simulink model "Devastator_simulator_2019a"  (R2019a)
settings: Solver=ode1  StartTime=0.0  StopTime=90  FixedStep=0.01  RelTol=1e-3
values from neighbouring files (symbols this model uses):
  Kd_psi = 0    [Devastator_simulator.m]
  Kd_Vx = 0    [Devastator_simulator.m]
  Ki_psi = 0    [Devastator_simulator.m]
  Ki_Vx = 1.85    [Devastator_simulator.m]
  Kp_psi = 0.4    [Devastator_simulator.m]
  Kp_Vx = 2    [Devastator_simulator.m]
  ox = str2num(x{6})    [Devastator_simulator.m]
  oy = str2num(x{7})    [Devastator_simulator.m]
  psi_0 = str2num(x{5})/180*pi    [Devastator_simulator.m]
  X_0 = str2num(x{3})    [Devastator_simulator.m]
  X_goal = str2num(x{1})    [Devastator_simulator.m]
  Y_0 = str2num(x{4})    [Devastator_simulator.m]
  Y_goal = str2num(x{2})    [Devastator_simulator.m]
libraries: simulink x4, slident x1
settings Model: Creator=PC  LastModifiedBy=PC

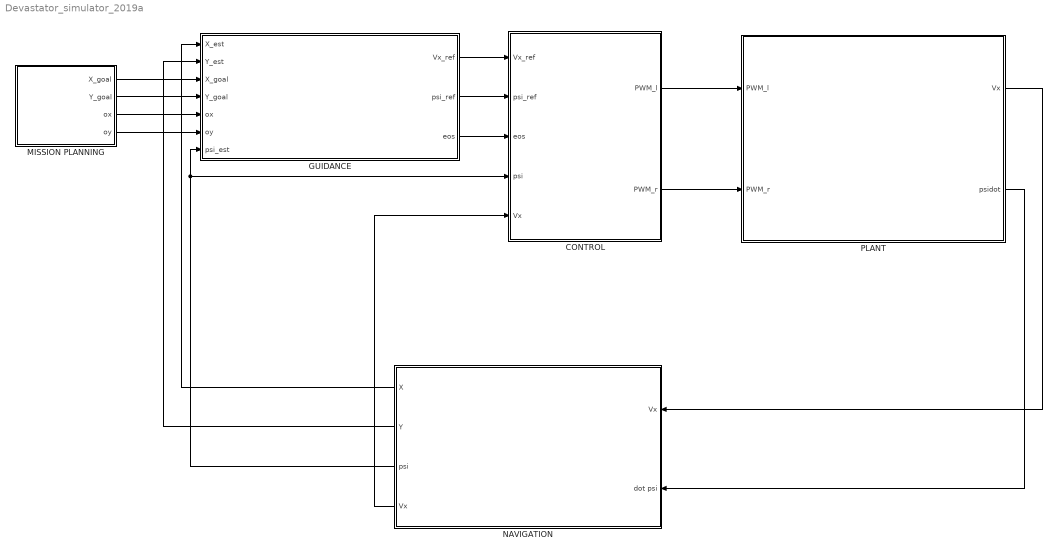
== system Devastator_simulator_2019a ==
  "CONTROL " : Subsystem
  "GUIDANCE " : Subsystem
  MISSION PLANNING : Subsystem
  NAVIGATION : Subsystem
  PLANT : Subsystem
  wires:
  "CONTROL "/1(PWM_l) -> PLANT/1(PWM_l)
  "CONTROL "/2(PWM_r) -> PLANT/2(PWM_r)
  PLANT/1(Vx) -> NAVIGATION/1(Vx)
  PLANT/2(psidot) -> NAVIGATION/2(dot psi)
  "GUIDANCE "/3(eos) -> "CONTROL "/3(eos)
  "GUIDANCE "/2(psi_ref) -> "CONTROL "/2(psi_ref)
  "GUIDANCE "/1(Vx_ref) -> "CONTROL "/1(Vx_ref)
  MISSION PLANNING/4(oy) -> "GUIDANCE "/6(oy)
  MISSION PLANNING/3(ox) -> "GUIDANCE "/5(ox)
  MISSION PLANNING/2(Y_goal) -> "GUIDANCE "/4(Y_goal)
  MISSION PLANNING/1(X_goal) -> "GUIDANCE "/3(X_goal)
  NAVIGATION/2(Y) -> "GUIDANCE "/2(Y_est)
  NAVIGATION/1(X) -> "GUIDANCE "/1(X_est)
  NAVIGATION/4(" Vx") -> "CONTROL "/5(Vx)
  NAVIGATION/3(psi) -> "GUIDANCE "/7(psi_est), "CONTROL "/4(psi)

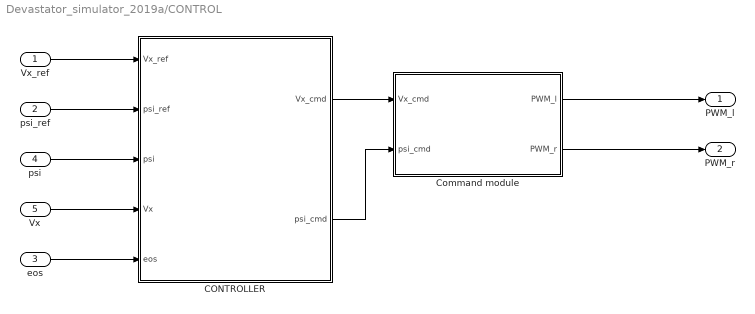
== system Devastator_simulator_2019a/CONTROL  ==
  Vx_ref : Inport
  psi_ref : Inport  Port=2
  eos : Inport  Port=3
  psi : Inport  Port=4
  Vx : Inport  Port=5
  CONTROLLER : Subsystem
  Command module : Subsystem
  PWM_l : Outport
  PWM_r : Outport  Port=2
  wires:
  psi_ref/1 -> CONTROLLER/2(psi_ref)
  eos/1 -> CONTROLLER/5(eos)
  psi/1 -> CONTROLLER/3(psi)
  CONTROLLER/1(Vx_cmd) -> Command module/1(Vx_cmd)
  CONTROLLER/2(psi_cmd) -> Command module/2(psi_cmd)
  Vx/1 -> CONTROLLER/4(Vx)
  Vx_ref/1 -> CONTROLLER/1(Vx_ref)
  Command module/1(PWM_l) -> PWM_l/1
  Command module/2(PWM_r) -> PWM_r/1

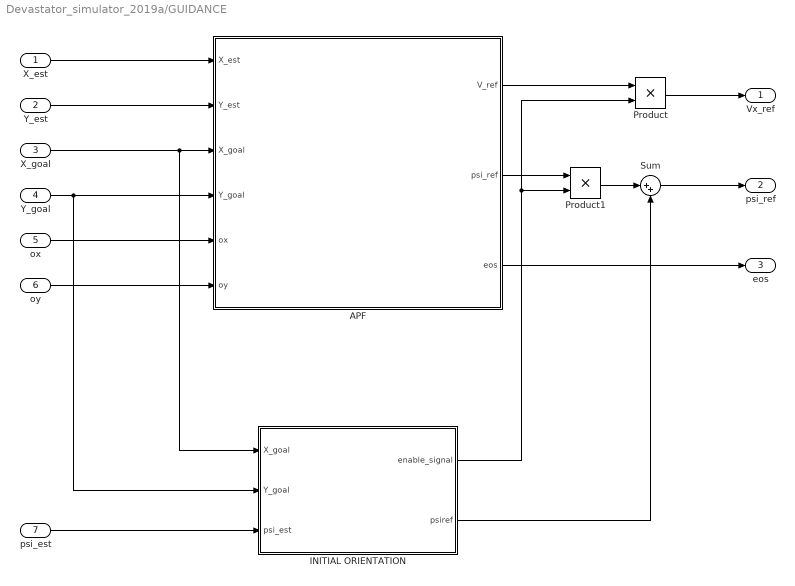
== system Devastator_simulator_2019a/GUIDANCE  ==
  X_est : Inport
  Y_est : Inport  Port=2
  X_goal : Inport  Port=3
  Y_goal : Inport  Port=4
  ox : Inport  Port=5
  oy : Inport  Port=6
  psi_est : Inport  Port=7
  APF : Subsystem
  INITIAL ORIENTATION : Subsystem
  Product : Product
  Product1 : Product
  Sum : Sum  Inputs=|++
  Vx_ref : Outport
  psi_ref : Outport  Port=2
  eos : Outport  Port=3
  wires:
  X_goal/1 -> INITIAL ORIENTATION/1(X_goal), APF/3(X_goal)
  Y_goal/1 -> INITIAL ORIENTATION/2(Y_goal), APF/4(Y_goal)
  X_est/1 -> APF/1(X_est)
  Y_est/1 -> APF/2(Y_est)
  ox/1 -> APF/5(ox)
  oy/1 -> APF/6(oy)
  Sum/1 -> psi_ref/1
  psi_est/1 -> INITIAL ORIENTATION/3(psi_est)
  INITIAL ORIENTATION/2(psiref) -> Sum/2
  APF/1(V_ref) -> Product/1
  Product/1 -> Vx_ref/1
  INITIAL ORIENTATION/1(enable_signal) -> Product1/2, Product/2
  APF/2(psi_ref) -> Product1/1
  Product1/1 -> Sum/1
  APF/3(eos) -> eos/1

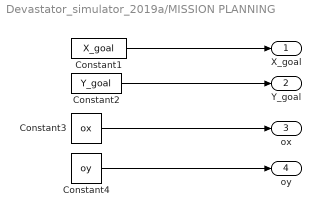
== system Devastator_simulator_2019a/MISSION PLANNING ==
  Constant1 : Constant  Value=X_goal
  Constant2 : Constant  Value=Y_goal
  Constant3 : Constant  Value=ox
  Constant4 : Constant  Value=oy
  X_goal : Outport
  Y_goal : Outport  Port=2
  ox : Outport  Port=3
  oy : Outport  Port=4
  wires:
  Constant4/1 -> oy/1
  Constant3/1 -> ox/1
  Constant2/1 -> Y_goal/1
  Constant1/1 -> X_goal/1

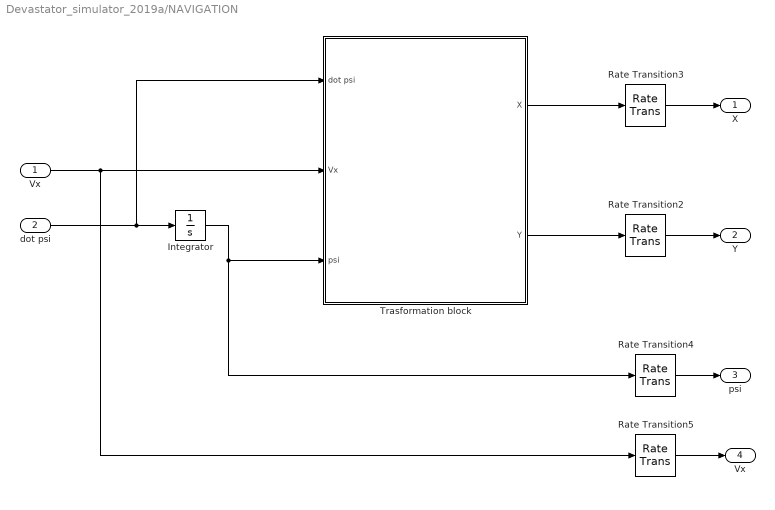
== system Devastator_simulator_2019a/NAVIGATION ==
  Vx : Inport
  dot psi : Inport  Port=2
  Integrator : Integrator  InitialCondition=psi_0  WrapState=on
  Rate Transition{2..5} (4 alike) : RateTransition  OutPortSampleTime=0.1
  Trasformation block : Subsystem
  X : Outport
  Y : Outport  Port=2
  psi : Outport  Port=3
  " Vx" : Outport  Port=4
  wires:
  dot psi/1 -> Trasformation block/1(dot psi), Integrator/1
  Rate Transition5/1 -> " Vx"/1
  Trasformation block/1(X) -> Rate Transition3/1
  Trasformation block/2(Y) -> Rate Transition2/1
  Rate Transition4/1 -> psi/1
  Rate Transition2/1 -> Y/1
  Vx/1 -> Rate Transition5/1, Trasformation block/2(Vx)
  Rate Transition3/1 -> X/1
  Integrator/1 -> Rate Transition4/1, Trasformation block/3(psi)

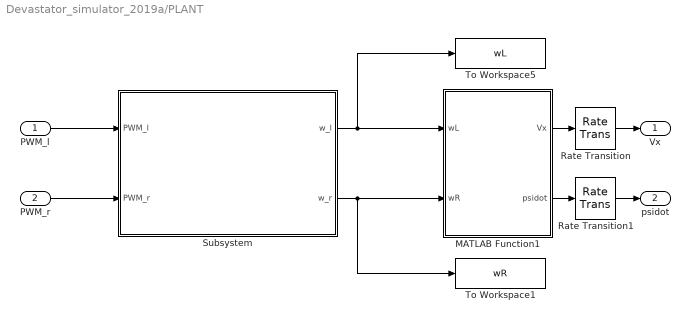
== system Devastator_simulator_2019a/PLANT ==
  PWM_l : Inport
  PWM_r : Inport  Port=2
  MATLAB Function1 : MATLAB Function  TreatAsAtomicUnit=on
  Rate Transition : RateTransition
  Rate Transition1 : RateTransition
  Subsystem : Subsystem
  To Workspace1 : ToWorkspace  VariableName=wR  SaveFormat=Structure With Time  SampleTime=-1
  To Workspace5 : ToWorkspace  VariableName=wL  SaveFormat=Structure With Time  SampleTime=-1
  Vx : Outport
  psidot : Outport  Port=2
  wires:
  MATLAB Function1/1(Vx) -> Rate Transition/1
  MATLAB Function1/2(psidot) -> Rate Transition1/1
  Subsystem/2(w_r) -> To Workspace1/1, MATLAB Function1/2(wR)
  Subsystem/1(w_l) -> To Workspace5/1, MATLAB Function1/1(wL)
  PWM_l/1 -> Subsystem/1(PWM_l)
  PWM_r/1 -> Subsystem/2(PWM_r)
  Rate Transition/1 -> Vx/1
  Rate Transition1/1 -> psidot/1

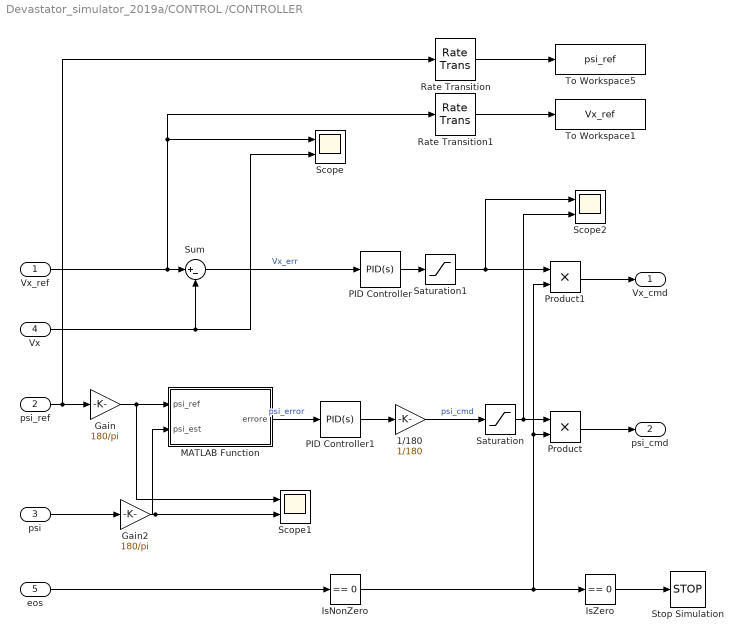
== system Devastator_simulator_2019a/CONTROL /CONTROLLER ==
  Vx_ref : Inport
  psi_ref : Inport  Port=2
  psi : Inport  Port=3
  Vx : Inport  Port=4
  eos : Inport  Port=5
  1/180 : Gain  Gain=1/180
  Gain : Gain  Gain=180/pi
  Gain2 : Gain  Gain=180/pi
  IsNonZero : simulink/Logic and Bit Operations/Compare To Zero  relop===  OutDataTypeStr=boolean
  IsZero : simulink/Logic and Bit Operations/Compare To Zero  relop===  OutDataTypeStr=boolean
  MATLAB Function : MATLAB Function  TreatAsAtomicUnit=on
  PID Controller : simulink/Continuous/PID Controller  Controller=PID  Form=Parallel  TimeDomain=Continuous-time  SampleTime=-1  IntegratorMethod=Forward Euler  FilterMethod=Forward Euler  ControllerParametersSource=internal  P=Kp_Vx  I=Ki_Vx  D=Kd_Vx  UseFilter=on  N=100  TunerSelectOption=Transfer Function Based (PID Tuner App)  InitialConditionSource=internal  InitialConditionForIntegrator=0  InitialConditionForFilter=0  DifferentiatorICPrevScaledInput=0  ExternalReset=none  TrackingMode=off  Kt=1  LimitOutput=off  UpperSaturationLimit=inf  LowerSaturationLimit=-inf  LinearizeAsGain=on  AntiWindupMode=none  Kb=1  POutMin=[]  POutMax=[]  IOutMin=[]  IOutMax=[]  DOutMin=[]  DOutMax=[]  NOutMin=[]  NOutMax=[]  SumOutMin=[]  SumOutMax=[]  SaturationOutMin=[]  SaturationOutMax=[]  PParamMin=[]  PParamMax=[]  IParamMin=[]  IParamMax=[]  DParamMin=[]  DParamMax=[]  NParamMin=[]  NParamMax=[]  KbParamMin=[]  KbParamMax=[]  KtParamMin=[]  KtParamMax=[]  KbOutMin=[]  KbOutMax=[]  KtOutMin=[]  KtOutMax=[]  IntegratorOutMin=[]  IntegratorOutMax=[]  FilterOutMin=[]  FilterOutMax=[]  SumI1OutMin=[]  SumI1OutMax=[]  SumI2OutMin=[]  SumI2OutMax=[]  SumI3OutMin=[]  SumI3OutMax=[]  SumI4OutMin=[]  SumI4OutMax=[]  SumDOutMin=[]  SumDOutMax=[]  DifferentiatorOutMin=[]  DifferentiatorOutMax=[]  FilterDiffOutCoefMin=[]  FilterDiffOutCoefMax=[]  ReciprocalOutMin=[]  ReciprocalOutMax=[]  SumDenOutMin=[]  SumDenOutMax=[]  SumNumOutMin=[]  SumNumOutMax=[]  DivideOutMin=[]  DivideOutMax=[]  IntegratorContinuousStateAttributes=''  IntegratorStateMustResolveToSignalObject=off  IntegratorRTWStateStorageClass=Auto  FilterContinuousStateAttributes=''  FilterStateMustResolveToSignalObject=off  FilterRTWStateStorageClass=Auto  ParallelPVariant=InternalParameters  IdealPVariant=Disabled  IVariant=InternalParameters  DVariant=InternalParameters  IntegratorVariant=Continuous  SatVariant=Disabled  AWVariant=Passthrough  PCopyVariant=Disabled  TRVariant=Disabled  FdbkBlocksVariant=Forward  IdealPFdbkVariant=Disabled  SatFdbkVariant=Disabled  DerivativeFilterVariant=ContFilter  NVariant=InternalParameters  NCopyVariant=Disabled  FilterICVariant=InternalICsFilter  IntegratorICVariant=InternalICs  ExternalResetVariant=Disabled  TRSumVariant=Passthrough  SumFdbkVariant=Disabled  SumVariant=Sum_PID
  PID Controller1 : simulink/Continuous/PID Controller  Controller=PID  Form=Parallel  TimeDomain=Continuous-time  SampleTime=-1  IntegratorMethod=Forward Euler  FilterMethod=Forward Euler  ControllerParametersSource=internal  P=Kp_psi  I=Ki_psi  D=Kd_psi  UseFilter=on  N=100  TunerSelectOption=Transfer Function Based (PID Tuner App)  InitialConditionSource=internal  InitialConditionForIntegrator=0  InitialConditionForFilter=0  DifferentiatorICPrevScaledInput=0  ExternalReset=none  TrackingMode=off  Kt=1  LimitOutput=off  UpperSaturationLimit=inf  LowerSaturationLimit=-inf  LinearizeAsGain=on  AntiWindupMode=none  Kb=1  POutMin=[]  POutMax=[]  IOutMin=[]  IOutMax=[]  DOutMin=[]  DOutMax=[]  NOutMin=[]  NOutMax=[]  SumOutMin=[]  SumOutMax=[]  SaturationOutMin=[]  SaturationOutMax=[]  PParamMin=[]  PParamMax=[]  IParamMin=[]  IParamMax=[]  DParamMin=[]  DParamMax=[]  NParamMin=[]  NParamMax=[]  KbParamMin=[]  KbParamMax=[]  KtParamMin=[]  KtParamMax=[]  KbOutMin=[]  KbOutMax=[]  KtOutMin=[]  KtOutMax=[]  IntegratorOutMin=[]  IntegratorOutMax=[]  FilterOutMin=[]  FilterOutMax=[]  SumI1OutMin=[]  SumI1OutMax=[]  SumI2OutMin=[]  SumI2OutMax=[]  SumI3OutMin=[]  SumI3OutMax=[]  SumI4OutMin=[]  SumI4OutMax=[]  SumDOutMin=[]  SumDOutMax=[]  DifferentiatorOutMin=[]  DifferentiatorOutMax=[]  FilterDiffOutCoefMin=[]  FilterDiffOutCoefMax=[]  ReciprocalOutMin=[]  ReciprocalOutMax=[]  SumDenOutMin=[]  SumDenOutMax=[]  SumNumOutMin=[]  SumNumOutMax=[]  DivideOutMin=[]  DivideOutMax=[]  IntegratorContinuousStateAttributes=''  IntegratorStateMustResolveToSignalObject=off  IntegratorRTWStateStorageClass=Auto  FilterContinuousStateAttributes=''  FilterStateMustResolveToSignalObject=off  FilterRTWStateStorageClass=Auto  ParallelPVariant=InternalParameters  IdealPVariant=Disabled  IVariant=InternalParameters  DVariant=InternalParameters  IntegratorVariant=Continuous  SatVariant=Disabled  AWVariant=Passthrough  PCopyVariant=Disabled  TRVariant=Disabled  FdbkBlocksVariant=Forward  IdealPFdbkVariant=Disabled  SatFdbkVariant=Disabled  DerivativeFilterVariant=ContFilter  NVariant=InternalParameters  NCopyVariant=Disabled  FilterICVariant=InternalICsFilter  IntegratorICVariant=InternalICs  ExternalResetVariant=Disabled  TRSumVariant=Passthrough  SumFdbkVariant=Disabled  SumVariant=Sum_PID
  Product : Product
  Product1 : Product
  Rate Transition : RateTransition
  Rate Transition1 : RateTransition
  Saturation : Saturate
  Saturation1 : Saturate  UpperLimit=1  LowerLimit=-1
  Scope : Scope  NumInputPorts=2
  Scope1 : Scope  NumInputPorts=2
  Scope2 : Scope  NumInputPorts=2
  Stop Simulation : Stop
  Sum : Sum  Inputs=|+-
  To Workspace1 : ToWorkspace  VariableName=Vx_ref  SaveFormat=Structure With Time  SampleTime=-1
  To Workspace5 : ToWorkspace  VariableName=psi_ref  SaveFormat=Structure With Time  SampleTime=-1
  Vx_cmd : Outport
  psi_cmd : Outport  Port=2
  wires:
  MATLAB Function/1(errore) -> PID Controller1/1  "psi_error"
  1/180/1 -> Saturation/1  "psi_cmd"
  PID Controller/1 -> Saturation1/1
  PID Controller1/1 -> 1/180/1
  Gain/1 -> Scope1/1, MATLAB Function/1(psi_ref)
  Vx_ref/1 -> Rate Transition1/1, Scope/1, Sum/1
  Vx/1 -> Scope/2, Sum/2
  Gain2/1 -> Scope1/2, MATLAB Function/2(psi_est)
  eos/1 -> IsNonZero/1
  Saturation/1 -> Scope2/2, Product/1
  Product/1 -> psi_cmd/1
  Saturation1/1 -> Scope2/1, Product1/1
  Product1/1 -> Vx_cmd/1
  IsNonZero/1 -> IsZero/1, Product1/2, Product/2
  IsZero/1 -> Stop Simulation/1
  psi_ref/1 -> Rate Transition/1, Gain/1
  psi/1 -> Gain2/1
  Rate Transition/1 -> To Workspace5/1
  Rate Transition1/1 -> To Workspace1/1
  Sum/1 -> PID Controller/1  "Vx_err"

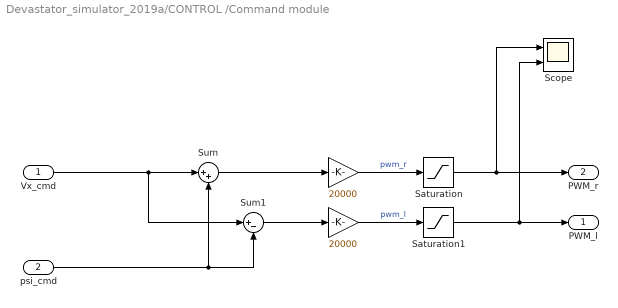
== system Devastator_simulator_2019a/CONTROL /Command module ==
  Vx_cmd : Inport
  psi_cmd : Inport  Port=2
  " " : Gain  Gain=20000
  "   " : Gain  Gain=20000
  Saturation : Saturate  UpperLimit=20000  LowerLimit=-20000
  Saturation1 : Saturate  UpperLimit=20000  LowerLimit=-20000
  Scope : Scope  NumInputPorts=2
  Sum : Sum  Inputs=|++
  Sum1 : Sum  Inputs=|+-
  PWM_l : Outport
  PWM_r : Outport  Port=2
  wires:
  "   "/1 -> Saturation1/1  "pwm_l"
  Sum1/1 -> "   "/1
  Vx_cmd/1 -> Sum/1, Sum1/1
  psi_cmd/1 -> Sum1/2, Sum/2
  Sum/1 -> " "/1
  " "/1 -> Saturation/1  "pwm_r"
  Saturation/1 -> Scope/1, PWM_r/1
  Saturation1/1 -> Scope/2, PWM_l/1

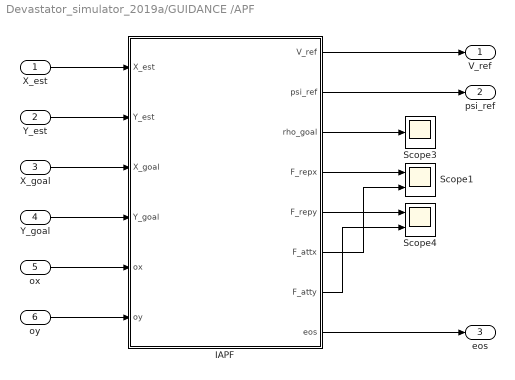
== system Devastator_simulator_2019a/GUIDANCE /APF ==
  X_est : Inport
  Y_est : Inport  Port=2
  X_goal : Inport  Port=3
  Y_goal : Inport  Port=4
  ox : Inport  Port=5
  oy : Inport  Port=6
  IAPF : MATLAB Function  TreatAsAtomicUnit=on
  Scope1 : Scope  NumInputPorts=2
  Scope3 : Scope
  Scope4 : Scope  NumInputPorts=2
  V_ref : Outport
  psi_ref : Outport  Port=2
  eos : Outport  Port=3
  wires:
  IAPF/1(V_ref) -> V_ref/1
  IAPF/6(F_attx) -> Scope1/2
  IAPF/3(rho_goal) -> Scope3/1
  IAPF/4(F_repx) -> Scope1/1
  IAPF/7(F_atty) -> Scope4/2
  IAPF/5(F_repy) -> Scope4/1
  X_est/1 -> IAPF/1(X_est)
  ox/1 -> IAPF/5(ox)
  IAPF/2(psi_ref) -> psi_ref/1
  Y_est/1 -> IAPF/2(Y_est)
  oy/1 -> IAPF/6(oy)
  IAPF/8(eos) -> eos/1
  X_goal/1 -> IAPF/3(X_goal)
  Y_goal/1 -> IAPF/4(Y_goal)

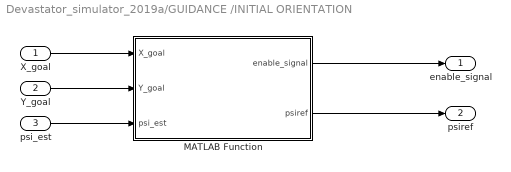
== system Devastator_simulator_2019a/GUIDANCE /INITIAL ORIENTATION ==
  X_goal : Inport
  Y_goal : Inport  Port=2
  psi_est : Inport  Port=3
  MATLAB Function : MATLAB Function  TreatAsAtomicUnit=on
  enable_signal : Outport
  psiref : Outport  Port=2
  wires:
  psi_est/1 -> MATLAB Function/3(psi_est)
  MATLAB Function/2(psiref) -> psiref/1
  Y_goal/1 -> MATLAB Function/2(Y_goal)
  X_goal/1 -> MATLAB Function/1(X_goal)
  MATLAB Function/1(enable_signal) -> enable_signal/1

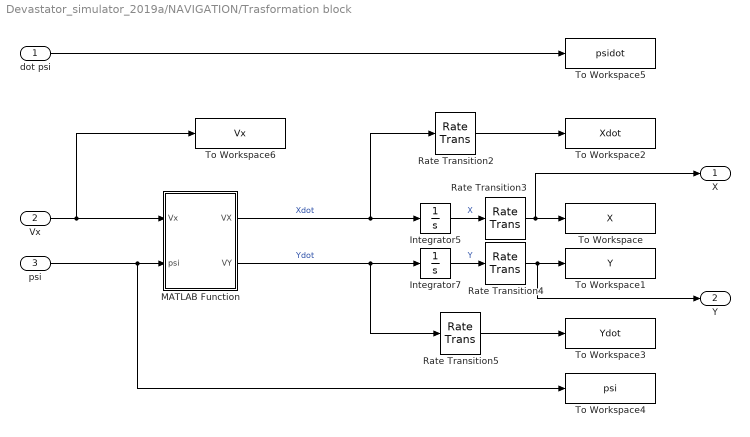
== system Devastator_simulator_2019a/NAVIGATION/Trasformation block ==
  dot psi : Inport
  Vx : Inport  Port=2
  psi : Inport  Port=3
  Integrator5 : Integrator  InitialCondition=X_0
  Integrator7 : Integrator  InitialCondition=Y_0
  MATLAB Function : MATLAB Function  TreatAsAtomicUnit=on
  Rate Transition{2..5} (4 alike) : RateTransition
  To Workspace : ToWorkspace  VariableName=X  SaveFormat=Structure With Time  SampleTime=-1
  To Workspace1 : ToWorkspace  VariableName=Y  SaveFormat=Structure With Time  SampleTime=-1
  To Workspace2 : ToWorkspace  VariableName=Xdot  SaveFormat=Structure With Time  SampleTime=-1
  To Workspace3 : ToWorkspace  VariableName=Ydot  SaveFormat=Structure With Time  SampleTime=-1
  To Workspace4 : ToWorkspace  VariableName=psi  SaveFormat=Structure With Time  SampleTime=-1
  To Workspace5 : ToWorkspace  VariableName=psidot  SaveFormat=Structure With Time  SampleTime=-1
  To Workspace6 : ToWorkspace  VariableName=Vx  SaveFormat=Structure With Time  SampleTime=-1
  X : Outport
  Y : Outport  Port=2
  wires:
  MATLAB Function/1(VX) -> Rate Transition2/1, Integrator5/1  "Xdot"
  Integrator7/1 -> Rate Transition4/1  "Y"
  MATLAB Function/2(VY) -> Rate Transition5/1, Integrator7/1  "Ydot"
  Integrator5/1 -> Rate Transition3/1  "X"
  dot psi/1 -> To Workspace5/1
  Vx/1 -> To Workspace6/1, MATLAB Function/1(Vx)
  Rate Transition2/1 -> To Workspace2/1
  Rate Transition3/1 -> X/1, To Workspace/1
  Rate Transition4/1 -> Y/1, To Workspace1/1
  Rate Transition5/1 -> To Workspace3/1
  psi/1 -> To Workspace4/1, MATLAB Function/2(psi)

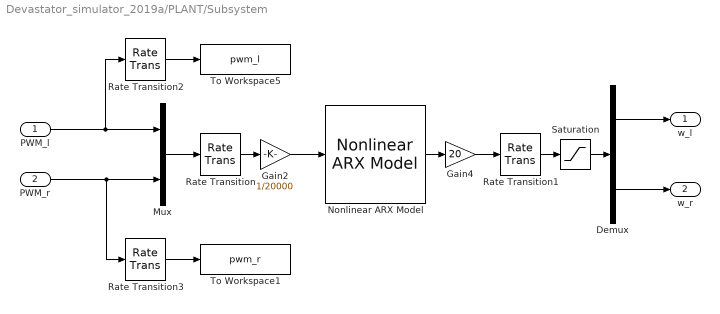
== system Devastator_simulator_2019a/PLANT/Subsystem ==
  PWM_l : Inport
  PWM_r : Inport  Port=2
  Demux : Demux  Outputs=2
  Gain2 : Gain  Gain=1/20000
  Gain4 : Gain  Gain=20
  Mux : Mux  Inputs=2
  Nonlinear ARX Model : slident/Models/Nonlinear ARX Model  sys=nlarx1  ICspec=Input and output values  X0=0  U0=0  Y0=0
      settings: SourceProductBaseCode=ID
  Rate Transition{,1..3} (4 alike) : RateTransition
  Saturation : Saturate  UpperLimit=20  LowerLimit=-20
  To Workspace1 : ToWorkspace  VariableName=pwm_r  SaveFormat=Structure With Time  SampleTime=-1
  To Workspace5 : ToWorkspace  VariableName=pwm_l  SaveFormat=Structure With Time  SampleTime=-1
  w_l : Outport
  w_r : Outport  Port=2
  wires:
  Demux/2 -> w_r/1
  Mux/1 -> Rate Transition/1
  PWM_l/1 -> Rate Transition2/1, Mux/1
  Rate Transition1/1 -> Saturation/1
  Nonlinear ARX Model/1 -> Gain4/1
  Gain2/1 -> Nonlinear ARX Model/1
  Rate Transition/1 -> Gain2/1
  Gain4/1 -> Rate Transition1/1
  Saturation/1 -> Demux/1
  Demux/1 -> w_l/1
  PWM_r/1 -> Rate Transition3/1, Mux/2
  Rate Transition2/1 -> To Workspace5/1
  Rate Transition3/1 -> To Workspace1/1

== matlab function Devastator_simulator_2019a/GUIDANCE /INITIAL ORIENTATION/MATLAB Function ==
  data: X_goal input; enable_signal output; Y_goal input; psi_est input; psiref output
function [enable_signal, psiref] = fcn(X_goal, Y_goal, psi_est)
psiref=0;
enable_signal=0;

persistent en
if isempty(en)
    en=0;
end

if en==0
if -pi<psi_est && psi_est<=-pi/2 
  if X_goal>=0 && Y_goal>=0
      enable_signal=0;
      psiref=0;
      en=0;
  end
   if X_goal>0 && Y_goal<0
      enable_signal=0;
      psiref=0;
      en=0;
   end
    if X_goal<=0 && Y_goal<=0
      enable_signal=1;
      en=1;
      psiref=0;
    end
    if X_goal<0 && Y_goal>0
      enable_signal=1;
      en=1;
      psiref=0;
    end
end
if pi/2<psi_est && psi_est<=pi 
  if X_goal>=0 && Y_goal>=0
      enable_signal=0;
      psiref=0;
      en=0;
  end
   if X_goal>0 && Y_goal<0
      enable_signal=0;
      psiref=0;
      en=0;
   end
    if X_goal<=0 && Y_goal<=0
      enable_signal=1;
      en=1;
      psiref=0;
    end
    if X_goal<0 && Y_goal>0
      enable_signal=1;
      en=1;
      psiref=0;
    end
end

if -pi/2<=psi_est && psi_est<=pi/2
  if X_goal>=0 && Y_goal>=0
      enable_signal=1;
      en=1;
      psiref=0;
  end
   if X_goal>0 && Y_goal<0
      enable_signal=1;
      en=1;
      psiref=0;
   end
    if X_goal<=0 && Y_goal<=0
      enable_signal=0;
      psiref=-pi;
      en=0;
    end
    if X_goal<0 && Y_goal>0
      enable_signal=0;
      psiref=pi;
      en=0;
    end
end
else
    enable_signal=1;
    psiref=0;
end

== matlab function Devastator_simulator_2019a/PLANT/MATLAB Function1 ==
  data: wL input; Vx output; wR input; psidot output
function [Vx, psidot] = fcn(wL, wR)
r=0.043/2;
B=0.185;

Vx=(wR+wL)*r/2;
psidot=(wR-wL)*r/B;

== matlab function Devastator_simulator_2019a/NAVIGATION/Trasformation block/MATLAB Function ==
  data: Vx input; VX output; psi input; VY output
function [VX, VY] = fcn(Vx, psi)

M=[cos(psi) -sin(psi); sin(psi) cos(psi)];

X=M*Vx;
VX=X(1);
VY=X(2);

== matlab function Devastator_simulator_2019a/CONTROL /CONTROLLER/MATLAB Function ==
  data: psi_ref input; errore output; psi_est input
function errore = fcn(psi_ref, psi_est)
errore=psi_ref-psi_est;

if abs(errore)>180
    errore=errore-360*sign(errore);
end

== matlab function Devastator_simulator_2019a/GUIDANCE /APF/IAPF ==
  data: X_est input; V_ref output; Y_est input; X_goal input; Y_goal input; ox input; oy input; psi_ref output; rho_goal output; F_repx output; F_repy output; F_attx output; F_atty output; eos output
function [V_ref, psi_ref, rho_goal, F_repx, F_repy, F_attx, F_atty, eos]  = fcn(X_est, Y_est, X_goal, Y_goal,  ox, oy)

% Potential field characteristics
rho_0=0.7;                   % Area of influence of obstacle  [m]
kp = 0.15;                   % Attractive pottential gain
eta = 0.05;                  % Repulsive potential gain

q=[X_est, Y_est]';           % Actual position [m]       
qg=[X_goal, Y_goal]';        % Goal position   [m]
rho_goal=norm(q-qg,2);       % Distance actual position-goal position
d=2;                         % Distance from goal, point of attractive field characteristic switching

% ATTRACTIVE
if rho_goal<=d
F_attx = -kp*(X_est-X_goal);
F_atty = -kp*(Y_est-Y_goal);
else    
F_attx = -kp*(X_est-X_goal)*d/rho_goal;
F_atty = -kp*(Y_est-Y_goal)*d/rho_goal;
end


% REPULSIVE
F_repx=0;
F_repy=0;
dmin=10000;
qc=[0 0]';
obst=0;

for k=1:length(ox)
    qc=[ox(k) oy(k)]';                          % Obstacle position [m]
    dq = norm(q-qc,2);                          % Distance actual position- obstacle position
     
    if dmin >= dq
        dmin = dq;
        min_ost = k;
        qc=[ox(min_ost) oy(min_ost)]';
        rho = norm(q-qc,2) ;                    % Distance with the nearest obstacle
        
        if rho<=rho_0                           % Inside obstacle area! Danger
           F_repx=eta*(1/rho - 1/rho_0)*1/(rho).^2*(X_est-ox(min_ost))/norm(q-qc,2);
           F_repy=eta*(1/rho - 1/rho_0)*1/(rho).^2*(Y_est-oy(min_ost))/norm(q-qc,2);  
           obst=1/rho;
        end
     
     end
end

% To find the goal if the obstacle is near
dob=0.3;
dgr=0.3;

if norm(qg-qc,2)<=dob && norm(q-qg,2)<=dgr
    F_totx=F_attx;
    F_toty=F_atty;
else
    F_totx = F_attx+F_repx;
    F_toty = F_atty+F_repy;
end

% Potential Force
F_tot=norm([F_totx,F_toty]);


% ORIENTATION REFERENCE SIGNAL
psi_ref=atan2(F_toty,F_totx);


% VELOCITY REFERENCE SIGNAL
% 1° prova per il campo di velocità
% V_ref=F_totx/F_tot*0.3;

% 2° prova per il campo di velocità
delta=0.4/rho_goal+obst;
V_ref= 0.3*2/(2+delta);

% END OF SIMULATION
if abs(rho_goal)<=0.05
    V_ref=0;
    psi_ref=0;
    eos=1;
else
    eos=0;
end

% Mathematical minimum
if F_tot==0
    psi_ref=0;
    V_ref=-0.3;
end
